simulink model "UnitTest_CodeGen"  (R2020a)
settings: Solver=ode1  StartTime=0.0  StopTime=inf  FixedStep=Ts_BigModel.Ts_base  MaxStep=Ts  RelTol=1e-3
undefined symbols (not defined in the file or in its folder): FLIGHT_PERF_PARAM_V10, FLIGHT_PERF_PARAM_V1000, TASK_PARAM_V10, TASK_PARAM_V1000
libraries: simulink x2
settings Model: Creator=sl  LastModifiedBy=Administrator
settings DataIOCC: SaveOutput=off  SaveTime=off
settings OptimizationCC: DefaultParameterBehavior=Inlined  EnhancedBackFolding=on  PassReuseOutputArgsAs=Individual arguments  ZeroExternalMemoryAtStartup=off  ZeroInternalMemoryAtStartup=off  OptimizeBlockOrder=speed  DifferentSizesBufferReuse=on  OptimizationCustomize=off  EfficientTunableParamExpr=on
settings DebuggingCC: InheritedTsInSrcMsg=none  ParameterPrecisionLossMsg=none  ParameterTunabilityLossMsg=error  UnconnectedInputMsg=none  UnconnectedOutputMsg=none  UnconnectedLineMsg=none
settings HardwareCC: ProdBitPerPointer=32  ProdBitPerSizeT=32  ProdBitPerPtrDiffT=32  ProdLargestAtomicInteger=Long  ProdLargestAtomicFloat=Double  ProdWordSize=32  ProdHWDeviceType=ARM Compatible->ARM Cortex
settings ModelReferenceCC: ParallelModelReferenceMATLABWorkerInit=Copy Base Workspace  ModelReferenceNumInstancesAllowed=Single
settings SFSimCC: MATLABDynamicMemAlloc=off
settings RTWCC: SystemTargetFile=ert.tlc  GenCodeOnly=on  PackageGeneratedCodeAndArtifacts=on  TemplateMakefile=ert_default_tmf  GenerateReport=on  IncludeHyperlinkInReport=on  LaunchReport=on  GenerateTraceInfo=on  GenerateTraceReport=on  GenerateTraceReportSl=on  GenerateTraceReportSf=on  GenerateTraceReportEml=on
settings CodeAppCC: ForceParamTrailComments=on  IgnoreCustomStorageClasses=off  MaxIdLength=48  OperatorAnnotations=on  SimulinkDataObjDesc=on  SFDataObjDesc=on  MATLABFcnDesc=on  InsertBlockDesc=on  MATLABSourceComments=on
settings ERTTargetCC: TargetLangStandard=C99 (ISO)  GenerateSampleERTMain=on  LogVarNameModifier=none  SupportVariableSizeSignals=on  InlinedParameterPlacement=NonHierarchical  ERTCustomFileTemplate=example_file_process.tlc  ERTFilePackagingFormat=Compact

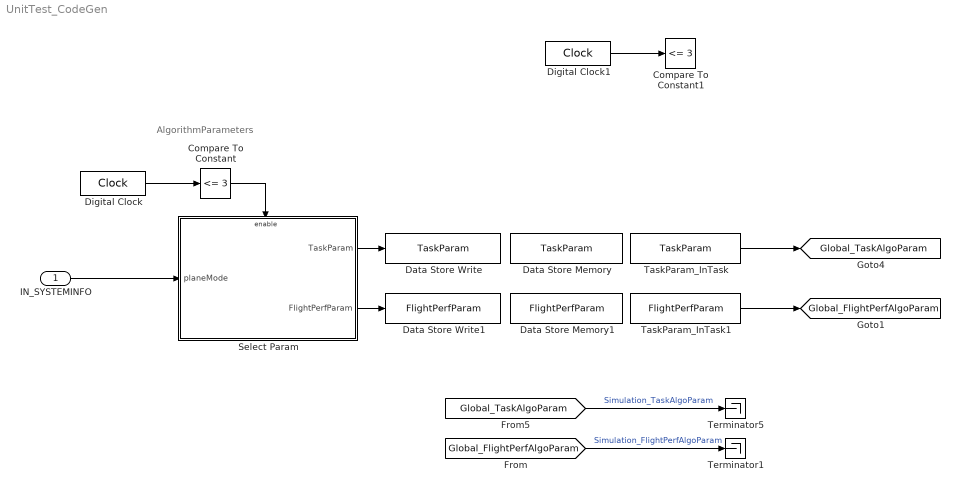
== system UnitTest_CodeGen ==
  note: AlgorithmParameters
  IN_SYSTEMINFO : Inport  OutDataTypeStr=Bus: BUS_SYSTEMINFO_INPUT  BusOutputAsStruct=on
  Compare To Constant : simulink/Logic and Bit Operations/Compare To Constant  relop=<=  const=3  OutDataTypeStr=boolean
  Compare To Constant1 : simulink/Logic and Bit Operations/Compare To Constant  relop=<=  const=3  OutDataTypeStr=boolean
  Data Store Memory : DataStoreMemory  DataStoreName=TaskParam  ReadBeforeWriteMsg=warning  WriteAfterWriteMsg=warning  WriteAfterReadMsg=warning  ShowAdditionalParam=off  OutDataTypeStr=Bus: BUS_TASK_PATH_AlgoParam  Dimensions=1
  Data Store Memory1 : DataStoreMemory  DataStoreName=FlightPerfParam  ReadBeforeWriteMsg=warning  WriteAfterWriteMsg=warning  WriteAfterReadMsg=warning  ShowAdditionalParam=off  OutDataTypeStr=Bus: BUS_FLIGHTPERF_PARAM  Dimensions=1
  Data Store Write : DataStoreWrite  DataStoreName=TaskParam
  Data Store Write1 : DataStoreWrite  DataStoreName=FlightPerfParam
  Digital Clock : DigitalClock  SampleTime=-1
  Digital Clock1 : DigitalClock  SampleTime=-1
  Select Param : Subsystem
  TaskParam_InTask : DataStoreRead  DataStoreName=TaskParam
  TaskParam_InTask1 : DataStoreRead  DataStoreName=FlightPerfParam
  Terminator1 : Terminator
  Terminator5 : Terminator
  tag scope: Global_FlightPerfAlgoParam=global, Global_TaskAlgoParam=global
  wires:
  Select Param/2(FlightPerfParam) -> Data Store Write1/1
  Select Param/1(TaskParam) -> Data Store Write/1
  TaskParam_InTask/1 -> [Global_TaskAlgoParam]
  IN_SYSTEMINFO/1 -> Select Param/1(planeMode)
  [Global_TaskAlgoParam] -> Terminator5/1  "Simulation_TaskAlgoParam"
  Digital Clock/1 -> Compare To Constant/1
  Compare To Constant/1 -> Select Param/Enable
  TaskParam_InTask1/1 -> [Global_FlightPerfAlgoParam]
  [Global_FlightPerfAlgoParam] -> Terminator1/1  "Simulation_FlightPerfAlgoParam"
  Digital Clock1/1 -> Compare To Constant1/1

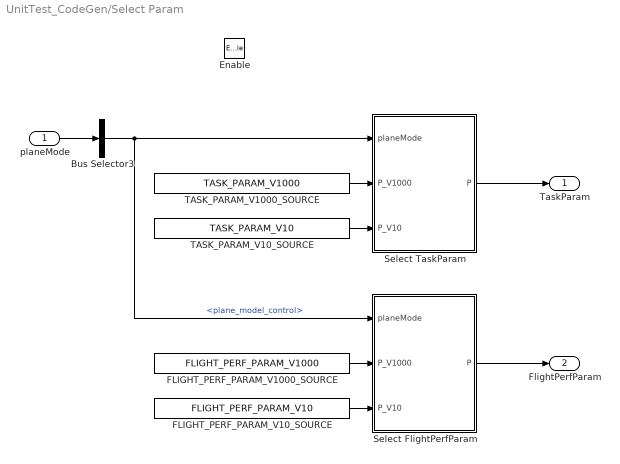
== system UnitTest_CodeGen/Select Param ==
  planeMode : Inport
  Enable : EnablePort
  Bus Selector3 : BusSelector  OutputSignals=plane_model_control
  FLIGHT_PERF_PARAM_V1000_SOURCE : Constant  Value=FLIGHT_PERF_PARAM_V1000  OutDataTypeStr=Bus: BUS_FLIGHTPERF_PARAM
  FLIGHT_PERF_PARAM_V10_SOURCE : Constant  Value=FLIGHT_PERF_PARAM_V10  OutDataTypeStr=Bus: BUS_FLIGHTPERF_PARAM
  Select FlightPerfParam : MATLAB Function  TreatAsAtomicUnit=on
  Select TaskParam : MATLAB Function  TreatAsAtomicUnit=on
  TASK_PARAM_V1000_SOURCE : Constant  Value=TASK_PARAM_V1000  OutDataTypeStr=Bus: BUS_TASK_PATH_AlgoParam
  TASK_PARAM_V10_SOURCE : Constant  Value=TASK_PARAM_V10  OutDataTypeStr=Bus: BUS_TASK_PATH_AlgoParam
  TaskParam : Outport
  FlightPerfParam : Outport  Port=2
  wires:
  TASK_PARAM_V1000_SOURCE/1 -> Select TaskParam/2(P_V1000)
  TASK_PARAM_V10_SOURCE/1 -> Select TaskParam/3(P_V10)
  Select TaskParam/1(P) -> TaskParam/1
  planeMode/1 -> Bus Selector3/1
  Bus Selector3/1 -> Select TaskParam/1(planeMode), Select FlightPerfParam/1(planeMode)  "<plane_model_control>"
  FLIGHT_PERF_PARAM_V10_SOURCE/1 -> Select FlightPerfParam/3(P_V10)
  FLIGHT_PERF_PARAM_V1000_SOURCE/1 -> Select FlightPerfParam/2(P_V1000)
  Select FlightPerfParam/1(P) -> FlightPerfParam/1

== matlab function UnitTest_CodeGen/Select Param/Select TaskParam ==
  data: planeMode input Enum: ENUM_plane_mode; P output Bus: BUS_TASK_PATH_AlgoParam; P_V1000 input Bus: BUS_TASK_PATH_AlgoParam; P_V10 input Bus: BUS_TASK_PATH_AlgoParam
function P = fcn(planeMode,P_V1000,P_V10)
switch planeMode
    case ENUM_plane_mode.V10
        P = P_V10;
    case {ENUM_plane_mode.V1000,ENUM_plane_mode.V10s}
        P = P_V1000;
    otherwise
        P = P_V1000;
end

== matlab function UnitTest_CodeGen/Select Param/Select FlightPerfParam ==
  data: planeMode input Enum: ENUM_plane_mode; P output Bus: BUS_FLIGHTPERF_PARAM; P_V1000 input Bus: BUS_FLIGHTPERF_PARAM; P_V10 input Bus: BUS_FLIGHTPERF_PARAM
function P = fcn(planeMode,P_V1000,P_V10)
switch planeMode
    case ENUM_plane_mode.V10
        P = P_V10;
    case {ENUM_plane_mode.V1000,ENUM_plane_mode.V10s}
        P = P_V1000;
    otherwise
        P = P_V1000;
end
